simulink model "PI_for_pumps_test"  (R2020a)
settings: Solver=FixedStepAuto  StartTime=0.0  StopTime=inf  FixedStep=1  RelTol=1e-3
libraries: modbusMatLib x6, simulink x4, realtime_pacer_lib x1
settings Model: Creator=pppc  LastModifiedBy=adish
settings DebuggingCC: InheritedTsInSrcMsg=none
settings SFSimCC: CustomCodeUndefinedFunction=UseInterfaceOnly

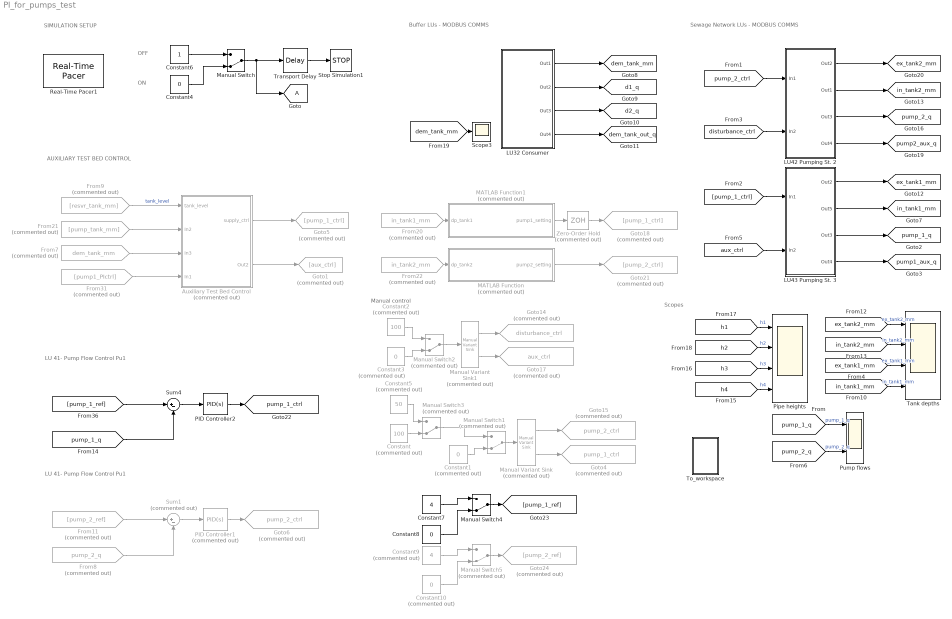
== system PI_for_pumps_test ==
  note: ON
  note: AUXILIARY TEST BED CONTROL
  note: OFF
  note: SIMULATION SETUP
  note: LU 41- Pump Flow Control Pu1
  note: Buffer LUs - MODBUS COMMS
  note: Sewage Network LUs - MODBUS COMMS
  note: Manual control
  note: Scopes
  note: LU 41- Pump Flow Control Pu1
  "Auxiliary Test Bed Control " : Subsystem  Commented=on
  Constant : Constant  Commented=on  Value=100
  Constant1 : Constant  Commented=on  Value=0
  Constant10 : Constant  Commented=on  Value=0
  Constant2 : Constant  Commented=on  Value=100
  Constant3 : Constant  Commented=on  Value=0
  Constant4 : Constant  Value=0
  Constant5 : Constant  Commented=on  Value=50
  Constant6 : Constant
  Constant7 : Constant  Value=4
  Constant8 : Constant  Value=0
  Constant9 : Constant  Commented=on  Value=4
  From11 : From  Commented=on  GotoTag=pump_2_ref
  From20 : From  Commented=on  GotoTag=in_tank1_mm  TagVisibility=global
  From21 : From  Commented=on  GotoTag=pump_tank_mm  TagVisibility=global
  From22 : From  Commented=on  GotoTag=in_tank2_mm  TagVisibility=global
  From31 : From  Commented=on  GotoTag=pump1_PIctrl  TagVisibility=global
  From7 : From  Commented=on  GotoTag=dem_tank_mm  TagVisibility=global
  From8 : From  Commented=on  GotoTag=pump_2_q  TagVisibility=global
  From9 : From  Commented=on  GotoTag=resvr_tank_mm  TagVisibility=global
  Goto1 : Goto  Commented=on  GotoTag=aux_ctrl
  Goto14 : Goto  Commented=on  GotoTag=disturbance_ctrl  TagVisibility=global
  Goto15 : Goto  Commented=on  GotoTag=pump_2_ctrl  TagVisibility=global
  Goto17 : Goto  Commented=on  GotoTag=aux_ctrl  TagVisibility=global
  Goto18 : Goto  Commented=on  GotoTag=pump_1_ctrl
  Goto21 : Goto  Commented=on  GotoTag=pump_2_ctrl
  Goto24 : Goto  Commented=on  GotoTag=pump_2_ref
  Goto4 : Goto  Commented=on  GotoTag=pump_1_ctrl  TagVisibility=global
  Goto5 : Goto  Commented=on  GotoTag=pump_1_ctrl
  Goto6 : Goto  Commented=on  GotoTag=pump_2_ctrl  TagVisibility=global
  LU32 Consumer : Subsystem
  LU42 Pumping St. 2 : Subsystem
  LU43 Pumping St. 3 : Subsystem
  MATLAB Function : MATLAB Function  Commented=on  TreatAsAtomicUnit=on
  MATLAB Function1 : MATLAB Function  Commented=on  TreatAsAtomicUnit=on
  Manual Variant Sink : simulink/Signal Routing/Manual Variant Sink  Commented=on  NumChoices=2  LabelModeActiveChoice=V_2
  Manual Variant Sink1 : simulink/Signal Routing/Manual Variant Sink  Commented=on  NumChoices=2  LabelModeActiveChoice=V_2
  Manual Switch : ManualSwitch  CurrentSetting=0
  Manual Switch{1..3,5} (4 alike) : ManualSwitch  Commented=on  CurrentSetting=0
  Manual Switch4 : ManualSwitch  CurrentSetting=0
  PID Controller1 : simulink/Continuous/PID Controller  Commented=on  Controller=PID  Form=Parallel  TimeDomain=Continuous-time  UseExternalTs=off  SampleTime=1  IntegratorMethod=Forward Euler  FilterMethod=Forward Euler  ControllerParametersSource=internal  P=7.4309  I=30.1148  D=0  UseFilter=on  N=100  TunerSelectOption=Transfer Function Based (PID Tuner App)  InitialConditionSource=internal  InitialConditionForIntegrator=0  InitialConditionForFilter=0  DifferentiatorICPrevScaledInput=0  ExternalReset=none  TrackingMode=off  Kt=1  LimitOutput=on  UpperSaturationLimit=95  LowerSaturationLimit=10  LinearizeAsGain=off  AntiWindupMode=clamping  Kb=1  POutMin=[]  POutMax=[]  IOutMin=[]  IOutMax=[]  DOutMin=[]  DOutMax=[]  NOutMin=[]  NOutMax=[]  SumOutMin=[]  SumOutMax=[]  SaturationOutMin=[]  SaturationOutMax=[]  PParamMin=[]  PParamMax=[]  IParamMin=[]  IParamMax=[]  DParamMin=[]  DParamMax=[]  NParamMin=[]  NParamMax=[]  KbParamMin=[]  KbParamMax=[]  KtParamMin=[]  KtParamMax=[]  KbOutMin=[]  KbOutMax=[]  KtOutMin=[]  KtOutMax=[]  IntegratorOutMin=[]  IntegratorOutMax=[]  FilterOutMin=[]  FilterOutMax=[]  SumI1OutMin=[]  SumI1OutMax=[]  SumI2OutMin=[]  SumI2OutMax=[]  SumI3OutMin=[]  SumI3OutMax=[]  SumI4OutMin=[]  SumI4OutMax=[]  SumDOutMin=[]  SumDOutMax=[]  DifferentiatorOutMin=[]  DifferentiatorOutMax=[]  FilterDiffOutCoefMin=[]  FilterDiffOutCoefMax=[]  ReciprocalOutMin=[]  ReciprocalOutMax=[]  SumDenOutMin=[]  SumDenOutMax=[]  SumNumOutMin=[]  SumNumOutMax=[]  DivideOutMin=[]  DivideOutMax=[]  UdiffTsProdOutMin=[]  UdiffTsProdOutMax=[]  NTsProdOutMin=[]  NTsProdOutMax=[]  UintegralTsProdOutMin=[]  UintegralTsProdOutMax=[]  UngainTsProdOutMin=[]  UngainTsProdOutMax=[]  IntegratorContinuousStateAttributes=''  IntegratorStateMustResolveToSignalObject=off  IntegratorRTWStateStorageClass=Auto  FilterContinuousStateAttributes=''  FilterStateMustResolveToSignalObject=off  FilterRTWStateStorageClass=Auto  ParallelPVariant=InternalParameters  IdealPVariant=Disabled  IVariant=InternalParameters  DVariant=InternalParameters  IntegratorVariant=Continuous  SatVariant=Enabled  AWVariant=ContClampingParallel  PCopyVariant=Disabled  TRVariant=Disabled  FdbkBlocksVariant=Forward  IdealPFdbkVariant=Disabled  SatFdbkVariant=Disabled  DerivativeFilterVariant=ContFilter  NVariant=InternalParameters  NCopyVariant=Disabled  FilterICVariant=InternalICsFilter  IntegratorICVariant=InternalICs  ExternalResetVariant=Disabled  TRSumVariant=Passthrough  SumFdbkVariant=Disabled  SumVariant=Sum_PID  TsampFilterVariant=InternalTs  TsampNgainVariant=Passthrough  TsampIntegralVariant=Passthrough
  PID Controller2 : simulink/Continuous/PID Controller  Controller=PID  Form=Parallel  TimeDomain=Continuous-time  UseExternalTs=off  SampleTime=1  IntegratorMethod=Forward Euler  FilterMethod=Forward Euler  ControllerParametersSource=internal  P=7.4309  I=30.1148  D=0  UseFilter=on  N=100  TunerSelectOption=Transfer Function Based (PID Tuner App)  InitialConditionSource=internal  InitialConditionForIntegrator=0  InitialConditionForFilter=0  DifferentiatorICPrevScaledInput=0  ExternalReset=none  TrackingMode=off  Kt=1  LimitOutput=on  UpperSaturationLimit=95  LowerSaturationLimit=10  LinearizeAsGain=off  AntiWindupMode=clamping  Kb=1  POutMin=[]  POutMax=[]  IOutMin=[]  IOutMax=[]  DOutMin=[]  DOutMax=[]  NOutMin=[]  NOutMax=[]  SumOutMin=[]  SumOutMax=[]  SaturationOutMin=[]  SaturationOutMax=[]  PParamMin=[]  PParamMax=[]  IParamMin=[]  IParamMax=[]  DParamMin=[]  DParamMax=[]  NParamMin=[]  NParamMax=[]  KbParamMin=[]  KbParamMax=[]  KtParamMin=[]  KtParamMax=[]  KbOutMin=[]  KbOutMax=[]  KtOutMin=[]  KtOutMax=[]  IntegratorOutMin=[]  IntegratorOutMax=[]  FilterOutMin=[]  FilterOutMax=[]  SumI1OutMin=[]  SumI1OutMax=[]  SumI2OutMin=[]  SumI2OutMax=[]  SumI3OutMin=[]  SumI3OutMax=[]  SumI4OutMin=[]  SumI4OutMax=[]  SumDOutMin=[]  SumDOutMax=[]  DifferentiatorOutMin=[]  DifferentiatorOutMax=[]  FilterDiffOutCoefMin=[]  FilterDiffOutCoefMax=[]  ReciprocalOutMin=[]  ReciprocalOutMax=[]  SumDenOutMin=[]  SumDenOutMax=[]  SumNumOutMin=[]  SumNumOutMax=[]  DivideOutMin=[]  DivideOutMax=[]  UdiffTsProdOutMin=[]  UdiffTsProdOutMax=[]  NTsProdOutMin=[]  NTsProdOutMax=[]  UintegralTsProdOutMin=[]  UintegralTsProdOutMax=[]  UngainTsProdOutMin=[]  UngainTsProdOutMax=[]  IntegratorContinuousStateAttributes=''  IntegratorStateMustResolveToSignalObject=off  IntegratorRTWStateStorageClass=Auto  FilterContinuousStateAttributes=''  FilterStateMustResolveToSignalObject=off  FilterRTWStateStorageClass=Auto  ParallelPVariant=InternalParameters  IdealPVariant=Disabled  IVariant=InternalParameters  DVariant=InternalParameters  IntegratorVariant=Continuous  SatVariant=Enabled  AWVariant=ContClampingParallel  PCopyVariant=Disabled  TRVariant=Disabled  FdbkBlocksVariant=Forward  IdealPFdbkVariant=Disabled  SatFdbkVariant=Disabled  DerivativeFilterVariant=ContFilter  NVariant=InternalParameters  NCopyVariant=Disabled  FilterICVariant=InternalICsFilter  IntegratorICVariant=InternalICs  ExternalResetVariant=Disabled  TRSumVariant=Passthrough  SumFdbkVariant=Disabled  SumVariant=Sum_PID  TsampFilterVariant=InternalTs  TsampNgainVariant=Passthrough  TsampIntegralVariant=Passthrough
  Pipe heights : Scope  NumInputPorts=4
  Pump flows : Scope  NumInputPorts=2
  Real-Time Pacer1 : realtime_pacer_lib/Real-Time Pacer  simTimePerRealTime=1
  Scope3 : Scope
  Stop Simulation1 : Stop
  Sum1 : Sum  Commented=on  Inputs=|+-
  Sum4 : Sum  Inputs=|+-
  Tank depths : Scope  NumInputPorts=4
  To_workspace : Subsystem
  Transport Delay : TransportDelay  DelayTime=2
  Zero-Order Hold : ZeroOrderHold  Commented=on  SampleTime=4
  tag scope: A=global, d1_q=global, d2_q=global, dem_tank_mm=global, dem_tank_out_q=global, ex_tank1_mm=global, ex_tank2_mm=global, in_tank1_mm=global, in_tank2_mm=global, pump1_aux_q=global, pump2_aux_q=global, pump_1_ctrl=global, pump_1_q=global, pump_2_q=global
  wires:
  Manual Switch/1 -> [A], Transport Delay/1
  Transport Delay/1 -> Stop Simulation1/1
  Constant6/1 -> Manual Switch/1
  Constant4/1 -> Manual Switch/2
  From9/1 -> "Auxiliary Test Bed Control "/1(tank_level)  "tank_level"
  From21/1 -> "Auxiliary Test Bed Control "/2(In2)
  From7/1 -> "Auxiliary Test Bed Control "/3(In3)
  "Auxiliary Test Bed Control "/1(supply_ctrl) -> Goto5/1
  "Auxiliary Test Bed Control "/2(Out2) -> Goto1/1
  LU32 Consumer/1(Out1) -> [dem_tank_mm]
  LU32 Consumer/2(Out2) -> [d1_q]
  LU32 Consumer/3(Out3) -> [d2_q]
  LU32 Consumer/4(Out4) -> [dem_tank_out_q]
  [pump_1_ref] -> Sum4/1
  [pump_1_q] -> Sum4/2
  Sum4/1 -> PID Controller2/1
  From31/1 -> "Auxiliary Test Bed Control "/4(In1)
  [pump_2_ctrl] -> LU42 Pumping St. 2/1(In1)
  LU42 Pumping St. 2/4(Out4) -> [pump2_aux_q]
  LU42 Pumping St. 2/1(Out2) -> [ex_tank2_mm]
  LU42 Pumping St. 2/3(Out3) -> [pump_2_q]
  [disturbance_ctrl] -> LU42 Pumping St. 2/2(In2)
  [aux_ctrl] -> LU43 Pumping St. 3/2(In2)
  LU43 Pumping St. 3/3(Out3) -> [pump_1_q]
  LU43 Pumping St. 3/4(Out4) -> [pump1_aux_q]
  [pump_1_ctrl] -> LU43 Pumping St. 3/1(In1)
  LU43 Pumping St. 3/1(Out2) -> [ex_tank1_mm]
  LU43 Pumping St. 3/2(Out5) -> [in_tank1_mm]
  Constant1/1 -> Manual Switch1/2
  Constant3/1 -> Manual Switch2/2
  Constant2/1 -> Manual Switch2/1
  Constant/1 -> Manual Switch3/2
  Constant5/1 -> Manual Switch3/1
  Manual Switch3/1 -> Manual Switch1/1
  LU42 Pumping St. 2/2(Out1) -> [in_tank2_mm]
  [in_tank2_mm] -> Tank depths/2  "in_tank2_mm"
  [ex_tank2_mm] -> Tank depths/1  "ex_tank2_mm"
  Manual Switch1/1 -> Manual Variant Sink/1
  Manual Variant Sink/1 -> Goto15/1
  Manual Variant Sink/2 -> Goto4/1
  Manual Switch2/1 -> Manual Variant Sink1/1
  Manual Variant Sink1/1 -> Goto14/1
  Manual Variant Sink1/2 -> Goto17/1
  [h1] -> Pipe heights/1  "h1"
  [h2] -> Pipe heights/2  "h2"
  [h4] -> Pipe heights/4  "h4"
  [h3] -> Pipe heights/3  "h3"
  [dem_tank_mm] -> Scope3/1
  MATLAB Function1/1(pump1_setting) -> Zero-Order Hold/1
  From20/1 -> MATLAB Function1/1(dp_tank1)
  Zero-Order Hold/1 -> Goto18/1
  From22/1 -> MATLAB Function/1(dp_tank2)
  MATLAB Function/1(pump2_setting) -> Goto21/1
  [ex_tank1_mm] -> Tank depths/3  "ex_tank1_mm"
  [in_tank1_mm] -> Tank depths/4  "in_tank1_mm"
  [pump_1_q] -> Pump flows/1  "pump_1_q"
  [pump_2_q] -> Pump flows/2  "pump_2_q"
  PID Controller2/1 -> [pump_1_ctrl]
  PID Controller1/1 -> Goto6/1
  Sum1/1 -> PID Controller1/1
  From8/1 -> Sum1/2
  From11/1 -> Sum1/1
  Manual Switch4/1 -> [pump_1_ref]
  Constant7/1 -> Manual Switch4/1
  Constant8/1 -> Manual Switch4/2
  Constant10/1 -> Manual Switch5/2
  Constant9/1 -> Manual Switch5/1
  Manual Switch5/1 -> Goto24/1

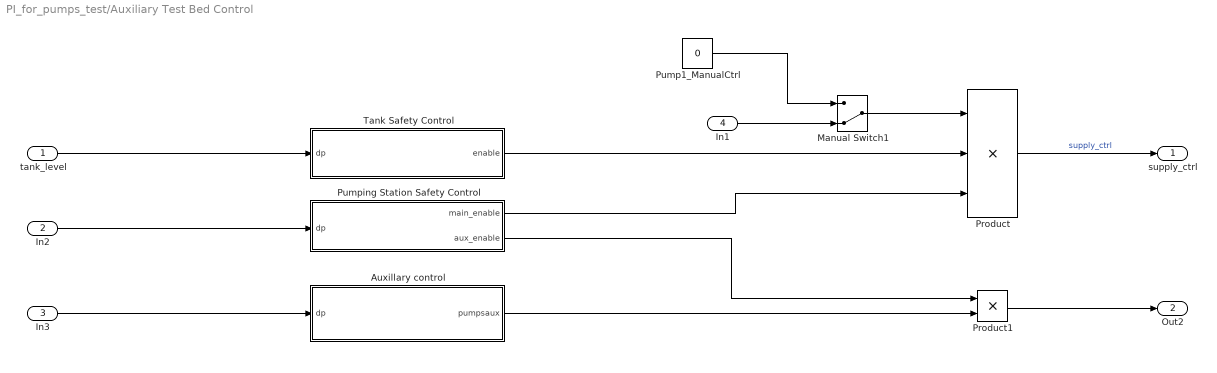
== system PI_for_pumps_test/Auxiliary Test Bed Control  ==
  tank_level : Inport
  In2 : Inport  Port=2
  In3 : Inport  Port=3
  In1 : Inport  Port=4
  Auxillary control : MATLAB Function  TreatAsAtomicUnit=on
  Manual Switch1 : ManualSwitch  CurrentSetting=0
  Product : Product  Inputs=3
  Product1 : Product
  Pump1_ManualCtrl : Constant  Value=0
  Pumping Station Safety Control : MATLAB Function  TreatAsAtomicUnit=on
  Tank Safety Control : MATLAB Function  TreatAsAtomicUnit=on
  supply_ctrl : Outport  VectorParamsAs1DForOutWhenUnconnected=off
  Out2 : Outport  Port=2  VectorParamsAs1DForOutWhenUnconnected=off
  wires:
  Pumping Station Safety Control/1(main_enable) -> Product/3
  Pump1_ManualCtrl/1 -> Manual Switch1/1
  Auxillary control/1(pumpsaux) -> Product1/2
  Tank Safety Control/1(enable) -> Product/2
  Pumping Station Safety Control/2(aux_enable) -> Product1/1
  Manual Switch1/1 -> Product/1
  Product1/1 -> Out2/1
  tank_level/1 -> Tank Safety Control/1(dp)
  In3/1 -> Auxillary control/1(dp)
  Product/1 -> supply_ctrl/1  "supply_ctrl"
  In2/1 -> Pumping Station Safety Control/1(dp)
  In1/1 -> Manual Switch1/2

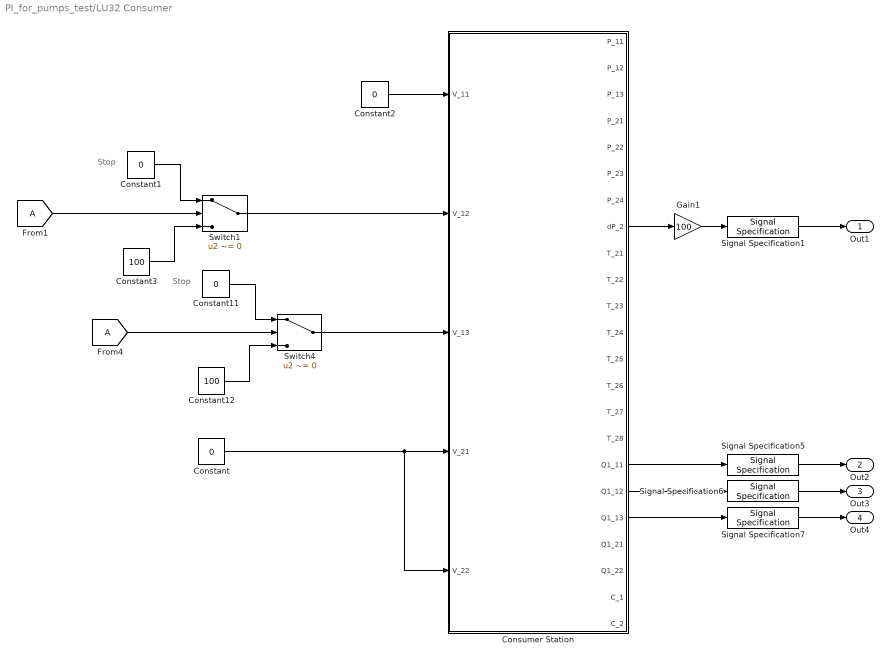
== system PI_for_pumps_test/LU32 Consumer ==
  note: Stop
  note: Stop
  Constant{,1..2,11} (4 alike) : Constant  Value=0
  Constant12 : Constant  Value=100
  Constant3 : Constant  Value=100
  Consumer Station : Subsystem
  Gain1 : Gain  Gain=100
  Signal Specification1 : SignalSpecification  Unit=mm
  Signal Specification5 : SignalSpecification  Unit=l/min
  Signal Specification6 : SignalSpecification  Unit=l/min
  Signal Specification7 : SignalSpecification  Unit=l/min
  Switch1 : Switch  Criteria=u2 ~= 0
  Switch4 : Switch  Criteria=u2 ~= 0
  Out1 : Outport  VectorParamsAs1DForOutWhenUnconnected=off
  Out2 : Outport  Port=2  VectorParamsAs1DForOutWhenUnconnected=off
  Out3 : Outport  Port=3  VectorParamsAs1DForOutWhenUnconnected=off
  Out4 : Outport  Port=4  VectorParamsAs1DForOutWhenUnconnected=off
  wires:
  Consumer Station/8(dP_2) -> Gain1/1
  Switch4/1 -> Consumer Station/3(V_13)
  Consumer Station/19(Q1_13) -> Signal Specification7/1
  Constant12/1 -> Switch4/3
  Consumer Station/17(Q1_11) -> Signal Specification5/1
  Consumer Station/18(Q1_12) -> Signal Specification6/1
  Gain1/1 -> Signal Specification1/1
  [A] -> Switch4/2
  Signal Specification7/1 -> Out4/1
  Constant11/1 -> Switch4/1
  Signal Specification5/1 -> Out2/1
  Constant/1 -> Consumer Station/5(V_22), Consumer Station/4(V_21)
  Signal Specification6/1 -> Out3/1
  Signal Specification1/1 -> Out1/1
  Constant1/1 -> Switch1/1
  [A] -> Switch1/2
  Constant3/1 -> Switch1/3
  Switch1/1 -> Consumer Station/2(V_12)
  Constant2/1 -> Consumer Station/1(V_11)

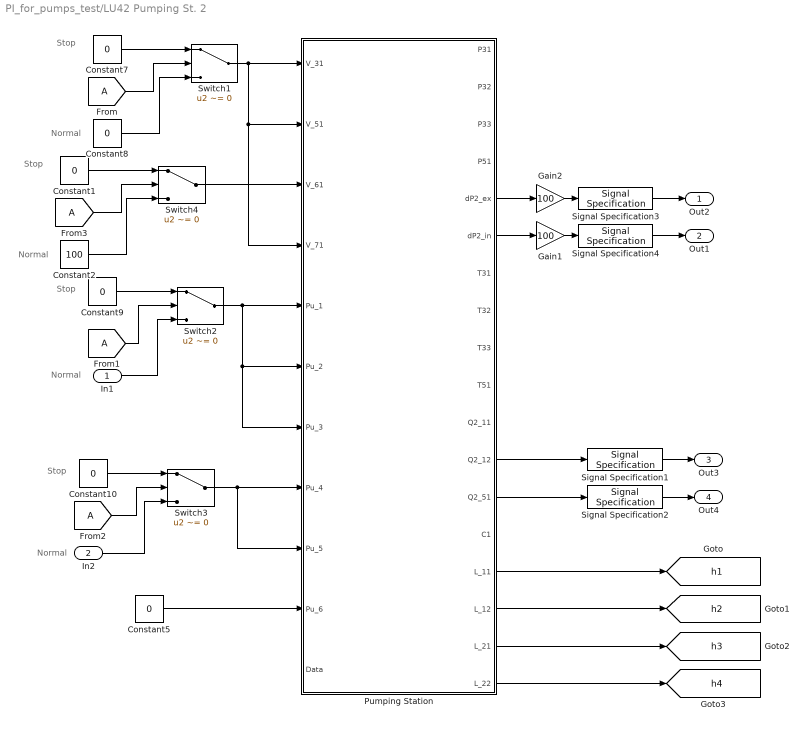
== system PI_for_pumps_test/LU42 Pumping St. 2 ==
  note: Stop
  note: Stop
  note: Normal
  note: Stop
  note: Normal
  note: Normal
  note: Stop
  note: Normal
  In1 : Inport
  In2 : Inport  Port=2
  Constant{1,5,7..10} (6 alike) : Constant  Value=0
  Constant2 : Constant  Value=100
  Gain1 : Gain  Gain=100
  Gain2 : Gain  Gain=100
  Pumping Station : Subsystem
  Signal Specification1 : SignalSpecification  Unit=l/min
  Signal Specification2 : SignalSpecification  Unit=l/min
  Signal Specification3 : SignalSpecification  Unit=mm
  Signal Specification4 : SignalSpecification  Unit=mm
  Switch{1..4} (4 alike) : Switch  Criteria=u2 ~= 0
  Out2 : Outport  VectorParamsAs1DForOutWhenUnconnected=off
  Out1 : Outport  Port=2  VectorParamsAs1DForOutWhenUnconnected=off
  Out3 : Outport  Port=3  VectorParamsAs1DForOutWhenUnconnected=off
  Out4 : Outport  Port=4  VectorParamsAs1DForOutWhenUnconnected=off
  tag scope: h1=global, h2=global, h3=global, h4=global
  wires:
  Switch2/1 -> Pumping Station/7(Pu_3), Pumping Station/6(Pu_2), Pumping Station/5(Pu_1)
  [A] -> Switch1/2
  Constant7/1 -> Switch1/1
  Constant8/1 -> Switch1/3
  Switch3/1 -> Pumping Station/9(Pu_5), Pumping Station/8(Pu_4)
  Constant10/1 -> Switch3/1
  In1/1 -> Switch2/3
  [A] -> Switch2/2
  Constant9/1 -> Switch2/1
  In2/1 -> Switch3/3
  Gain2/1 -> Signal Specification3/1
  Constant5/1 -> Pumping Station/10(Pu_6)
  Signal Specification3/1 -> Out2/1
  [A] -> Switch3/2
  Pumping Station/5(dP2_ex) -> Gain2/1
  Switch1/1 -> Pumping Station/4(V_71), Pumping Station/2(V_51), Pumping Station/1(V_31)
  Signal Specification1/1 -> Out3/1
  Signal Specification2/1 -> Out4/1
  Pumping Station/12(Q2_12) -> Signal Specification1/1
  Pumping Station/13(Q2_51) -> Signal Specification2/1
  Pumping Station/6(dP2_in) -> Gain1/1
  Gain1/1 -> Signal Specification4/1
  Signal Specification4/1 -> Out1/1
  Pumping Station/15(L_11) -> [h1]
  Pumping Station/16(L_12) -> [h2]
  Pumping Station/17(L_21) -> [h3]
  Pumping Station/18(L_22) -> [h4]
  Constant1/1 -> Switch4/1
  Constant2/1 -> Switch4/3
  [A] -> Switch4/2
  Switch4/1 -> Pumping Station/3(V_61)

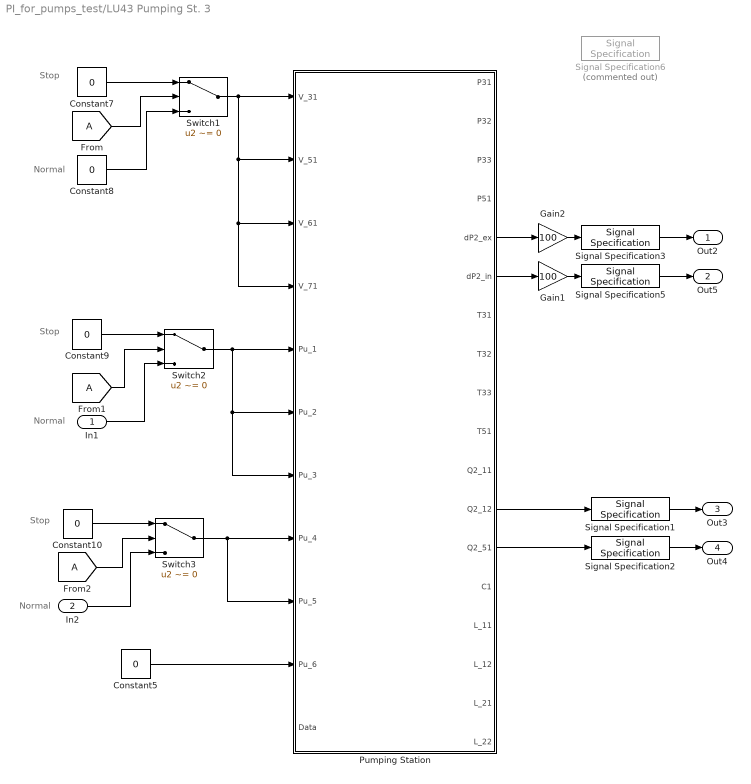
== system PI_for_pumps_test/LU43 Pumping St. 3 ==
  note: Stop
  note: Stop
  note: Normal
  note: Stop
  note: Normal
  note: Normal
  In1 : Inport
  In2 : Inport  Port=2
  Constant{5,7..10} (5 alike) : Constant  Value=0
  Gain1 : Gain  Gain=100
  Gain2 : Gain  Gain=100
  Pumping Station : Subsystem
  Signal Specification1 : SignalSpecification  Unit=l/min
  Signal Specification2 : SignalSpecification  Unit=l/min
  Signal Specification3 : SignalSpecification  Unit=mm
  Signal Specification5 : SignalSpecification  Unit=mm
  Signal Specification6 : SignalSpecification  Commented=on  Unit=bar
  Switch1 : Switch  Criteria=u2 ~= 0
  Switch2 : Switch  Criteria=u2 ~= 0
  Switch3 : Switch  Criteria=u2 ~= 0
  Out2 : Outport  VectorParamsAs1DForOutWhenUnconnected=off
  Out5 : Outport  Port=2  VectorParamsAs1DForOutWhenUnconnected=off
  Out3 : Outport  Port=3  VectorParamsAs1DForOutWhenUnconnected=off
  Out4 : Outport  Port=4  VectorParamsAs1DForOutWhenUnconnected=off
  wires:
  Switch2/1 -> Pumping Station/7(Pu_3), Pumping Station/6(Pu_2), Pumping Station/5(Pu_1)
  [A] -> Switch1/2
  Constant7/1 -> Switch1/1
  Constant8/1 -> Switch1/3
  Switch3/1 -> Pumping Station/9(Pu_5), Pumping Station/8(Pu_4)
  Constant10/1 -> Switch3/1
  In1/1 -> Switch2/3
  [A] -> Switch2/2
  Constant9/1 -> Switch2/1
  In2/1 -> Switch3/3
  Gain2/1 -> Signal Specification3/1
  Constant5/1 -> Pumping Station/10(Pu_6)
  Signal Specification3/1 -> Out2/1
  [A] -> Switch3/2
  Pumping Station/5(dP2_ex) -> Gain2/1
  Switch1/1 -> Pumping Station/4(V_71), Pumping Station/3(V_61), Pumping Station/2(V_51), Pumping Station/1(V_31)
  Signal Specification1/1 -> Out3/1
  Signal Specification2/1 -> Out4/1
  Pumping Station/12(Q2_12) -> Signal Specification1/1
  Pumping Station/13(Q2_51) -> Signal Specification2/1
  Pumping Station/6(dP2_in) -> Gain1/1
  Signal Specification5/1 -> Out5/1
  Gain1/1 -> Signal Specification5/1

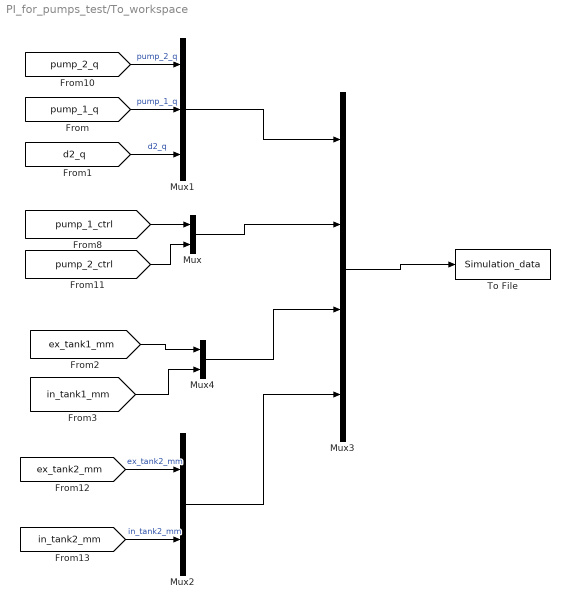
== system PI_for_pumps_test/To_workspace ==
  Mux : Mux  Inputs=2
  Mux1 : Mux  Inputs=3
  Mux2 : Mux  Inputs=2
  Mux3 : Mux
  Mux4 : Mux  Inputs=2
  To File : ToFile  Filename=Simulation_data  SaveFormat=Timeseries
  wires:
  [pump_2_q] -> Mux1/1  "pump_2_q"
  [in_tank2_mm] -> Mux2/2  "in_tank2_mm"
  [ex_tank2_mm] -> Mux2/1  "ex_tank2_mm"
  [pump_1_q] -> Mux1/2  "pump_1_q"
  [d2_q] -> Mux1/3  "d2_q"
  Mux1/1 -> Mux3/1
  Mux3/1 -> To File/1
  [pump_1_ctrl] -> Mux/1
  [pump_2_ctrl] -> Mux/2
  Mux/1 -> Mux3/2
  Mux2/1 -> Mux3/4
  [ex_tank1_mm] -> Mux4/1
  [in_tank1_mm] -> Mux4/2
  Mux4/1 -> Mux3/3

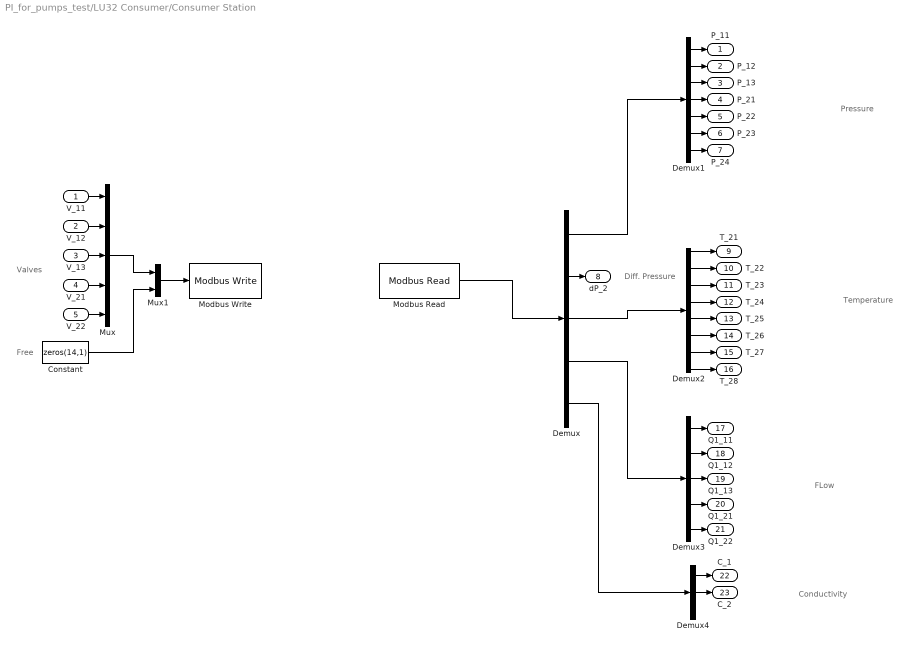
== system PI_for_pumps_test/LU32 Consumer/Consumer Station ==
  note: Pressure
  note: Temperature
  note: FLow
  note: Conductivity
  note: Valves
  note: Diff. Pressure
  note: Free
  V_11 : Inport
  V_12 : Inport  Port=2
  V_13 : Inport  Port=3
  V_21 : Inport  Port=4
  V_22 : Inport  Port=5
  Constant : Constant  Value=zeros(14,1)
  Demux : Demux  Outputs=[7 1 8 5 3]
  Demux1 : Demux  Outputs=7
  Demux2 : Demux  Outputs=8
  Demux3 : Demux  Outputs=5
  Demux4 : Demux  Outputs=3
  Modbus Read : modbusMatLib/Modbus Read  registry=0  ipAddress='192.168.100.32'  port=502
  Modbus Write : modbusMatLib/Modbus Write  registry=001  port=502  ipAddress='192.168.100.32'
  Mux : Mux  Inputs=5
  Mux1 : Mux  Inputs=2
  P_11 : Outport  VectorParamsAs1DForOutWhenUnconnected=off
  P_12 : Outport  Port=2  VectorParamsAs1DForOutWhenUnconnected=off
  P_13 : Outport  Port=3  VectorParamsAs1DForOutWhenUnconnected=off
  P_21 : Outport  Port=4  VectorParamsAs1DForOutWhenUnconnected=off
  P_22 : Outport  Port=5  VectorParamsAs1DForOutWhenUnconnected=off
  P_23 : Outport  Port=6  VectorParamsAs1DForOutWhenUnconnected=off
  P_24 : Outport  Port=7  VectorParamsAs1DForOutWhenUnconnected=off
  dP_2 : Outport  Port=8  VectorParamsAs1DForOutWhenUnconnected=off
  T_21 : Outport  Port=9  VectorParamsAs1DForOutWhenUnconnected=off
  T_22 : Outport  Port=10  VectorParamsAs1DForOutWhenUnconnected=off
  T_23 : Outport  Port=11  VectorParamsAs1DForOutWhenUnconnected=off
  T_24 : Outport  Port=12  VectorParamsAs1DForOutWhenUnconnected=off
  T_25 : Outport  Port=13  VectorParamsAs1DForOutWhenUnconnected=off
  T_26 : Outport  Port=14  VectorParamsAs1DForOutWhenUnconnected=off
  T_27 : Outport  Port=15  VectorParamsAs1DForOutWhenUnconnected=off
  T_28 : Outport  Port=16  VectorParamsAs1DForOutWhenUnconnected=off
  Q1_11 : Outport  Port=17  VectorParamsAs1DForOutWhenUnconnected=off
  Q1_12 : Outport  Port=18  VectorParamsAs1DForOutWhenUnconnected=off
  Q1_13 : Outport  Port=19  VectorParamsAs1DForOutWhenUnconnected=off
  Q1_21 : Outport  Port=20  VectorParamsAs1DForOutWhenUnconnected=off
  Q1_22 : Outport  Port=21  VectorParamsAs1DForOutWhenUnconnected=off
  C_1 : Outport  Port=22  VectorParamsAs1DForOutWhenUnconnected=off
  C_2 : Outport  Port=23  VectorParamsAs1DForOutWhenUnconnected=off
  wires:
  Mux/1 -> Mux1/1
  Mux1/1 -> Modbus Write/1
  Constant/1 -> Mux1/2
  Demux1/5 -> P_22/1
  V_12/1 -> Mux/2
  Demux1/6 -> P_23/1
  Demux1/3 -> P_13/1
  Demux1/4 -> P_21/1
  V_13/1 -> Mux/3
  Demux3/2 -> Q1_12/1
  Demux3/5 -> Q1_22/1
  Demux/2 -> dP_2/1
  Demux3/1 -> Q1_11/1
  Demux1/2 -> P_12/1
  Demux2/5 -> T_25/1
  Demux4/1 -> C_1/1
  V_21/1 -> Mux/4
  Demux3/3 -> Q1_13/1
  Demux1/1 -> P_11/1
  Demux3/4 -> Q1_21/1
  V_11/1 -> Mux/1
  Demux2/4 -> T_24/1
  Demux2/3 -> T_23/1
  Demux2/2 -> T_22/1
  Demux2/1 -> T_21/1
  Demux1/7 -> P_24/1
  V_22/1 -> Mux/5
  Demux2/7 -> T_27/1
  Demux/5 -> Demux4/1
  Demux/1 -> Demux1/1
  Demux2/8 -> T_28/1
  Demux4/2 -> C_2/1
  Demux/3 -> Demux2/1
  Demux/4 -> Demux3/1
  Modbus Read/1 -> Demux/1
  Demux2/6 -> T_26/1

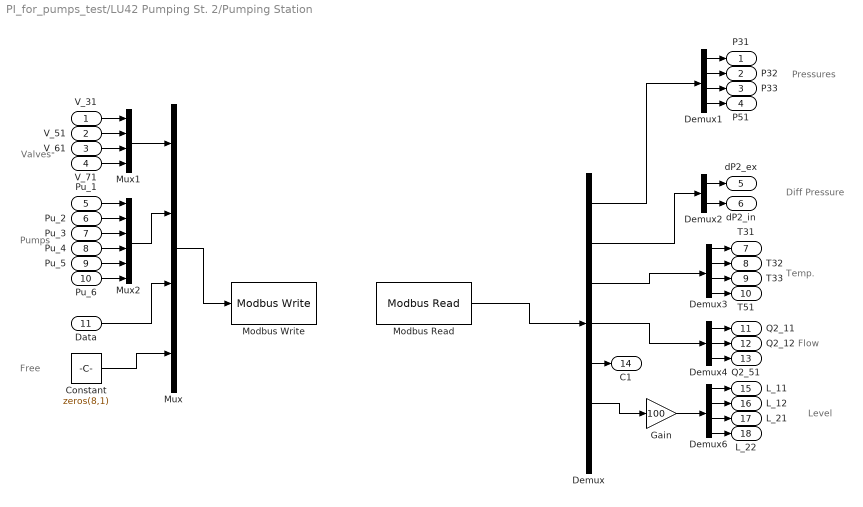
== system PI_for_pumps_test/LU42 Pumping St. 2/Pumping Station ==
  note: Free
  note: Pumps
  note: Valves
  note: Flow
  note: Temp.
  note: Diff Pressure
  note: Pressures
  note: Level
  V_31 : Inport
  V_51 : Inport  Port=2
  V_61 : Inport  Port=3
  V_71 : Inport  Port=4
  Pu_1 : Inport  Port=5
  Pu_2 : Inport  Port=6
  Pu_3 : Inport  Port=7
  Pu_4 : Inport  Port=8
  Pu_5 : Inport  Port=9
  Pu_6 : Inport  Port=10
  Data : Inport  Port=11
  Constant : Constant  Value=zeros(8,1)
  Demux : Demux  Outputs=[4 2 4 3 1 4 6]
  Demux1 : Demux
  Demux2 : Demux  Outputs=2
  Demux3 : Demux
  Demux4 : Demux  Outputs=3
  Demux6 : Demux
  Gain : Gain  Gain=100
  Modbus Read : modbusMatLib/Modbus Read  registry=0  ipAddress='192.168.100.42'  port=502
  Modbus Write : modbusMatLib/Modbus Write  registry=001  port=502  ipAddress='192.168.100.42'
  Mux : Mux
  Mux1 : Mux
  Mux2 : Mux  Inputs=6
  P31 : Outport  VectorParamsAs1DForOutWhenUnconnected=off
  P32 : Outport  Port=2  VectorParamsAs1DForOutWhenUnconnected=off
  P33 : Outport  Port=3  VectorParamsAs1DForOutWhenUnconnected=off
  P51 : Outport  Port=4  VectorParamsAs1DForOutWhenUnconnected=off
  dP2_ex : Outport  Port=5  VectorParamsAs1DForOutWhenUnconnected=off
  dP2_in : Outport  Port=6  VectorParamsAs1DForOutWhenUnconnected=off
  T31 : Outport  Port=7  VectorParamsAs1DForOutWhenUnconnected=off
  T32 : Outport  Port=8  VectorParamsAs1DForOutWhenUnconnected=off
  T33 : Outport  Port=9  VectorParamsAs1DForOutWhenUnconnected=off
  T51 : Outport  Port=10  VectorParamsAs1DForOutWhenUnconnected=off
  Q2_11 : Outport  Port=11  VectorParamsAs1DForOutWhenUnconnected=off
  Q2_12 : Outport  Port=12  VectorParamsAs1DForOutWhenUnconnected=off
  Q2_51 : Outport  Port=13  VectorParamsAs1DForOutWhenUnconnected=off
  C1 : Outport  Port=14  VectorParamsAs1DForOutWhenUnconnected=off
  L_11 : Outport  Port=15  VectorParamsAs1DForOutWhenUnconnected=off
  L_12 : Outport  Port=16  VectorParamsAs1DForOutWhenUnconnected=off
  L_21 : Outport  Port=17  VectorParamsAs1DForOutWhenUnconnected=off
  L_22 : Outport  Port=18  VectorParamsAs1DForOutWhenUnconnected=off
  wires:
  Demux4/1 -> Q2_11/1
  Demux/2 -> Demux2/1
  Demux/4 -> Demux4/1
  Demux2/1 -> dP2_ex/1
  Demux/3 -> Demux3/1
  Demux/1 -> Demux1/1
  Demux3/4 -> T51/1
  Demux1/4 -> P51/1
  Demux3/2 -> T32/1
  Modbus Read/1 -> Demux/1
  Demux6/1 -> L_11/1
  Demux6/2 -> L_12/1
  Demux4/3 -> Q2_51/1
  Demux4/2 -> Q2_12/1
  Demux6/3 -> L_21/1
  Demux6/4 -> L_22/1
  Demux3/3 -> T33/1
  Demux1/1 -> P31/1
  Demux1/2 -> P32/1
  Demux/5 -> C1/1
  Demux1/3 -> P33/1
  Demux2/2 -> dP2_in/1
  Demux3/1 -> T31/1
  Mux/1 -> Modbus Write/1
  Mux1/1 -> Mux/1
  V_31/1 -> Mux1/1
  V_51/1 -> Mux1/2
  V_61/1 -> Mux1/3
  V_71/1 -> Mux1/4
  Pu_4/1 -> Mux2/4
  Pu_3/1 -> Mux2/3
  Pu_1/1 -> Mux2/1
  Pu_2/1 -> Mux2/2
  Mux2/1 -> Mux/2
  Pu_5/1 -> Mux2/5
  Pu_6/1 -> Mux2/6
  Data/1 -> Mux/3
  Constant/1 -> Mux/4
  Gain/1 -> Demux6/1
  Demux/6 -> Gain/1

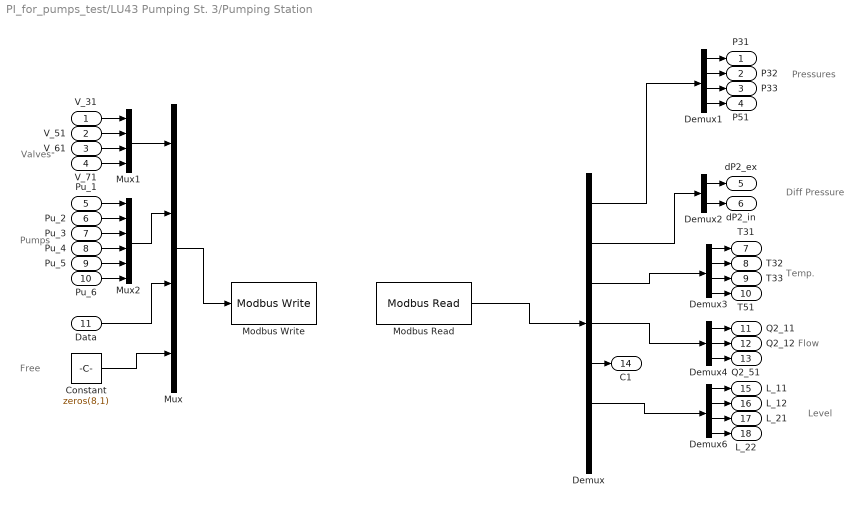
== system PI_for_pumps_test/LU43 Pumping St. 3/Pumping Station ==
  note: Free
  note: Pumps
  note: Valves
  note: Flow
  note: Temp.
  note: Diff Pressure
  note: Pressures
  note: Level
  V_31 : Inport
  V_51 : Inport  Port=2
  V_61 : Inport  Port=3
  V_71 : Inport  Port=4
  Pu_1 : Inport  Port=5
  Pu_2 : Inport  Port=6
  Pu_3 : Inport  Port=7
  Pu_4 : Inport  Port=8
  Pu_5 : Inport  Port=9
  Pu_6 : Inport  Port=10
  Data : Inport  Port=11
  Constant : Constant  Value=zeros(8,1)
  Demux : Demux  Outputs=[4 2 4 3 1 4 6]
  Demux1 : Demux
  Demux2 : Demux  Outputs=2
  Demux3 : Demux
  Demux4 : Demux  Outputs=3
  Demux6 : Demux
  Modbus Read : modbusMatLib/Modbus Read  registry=0  ipAddress='192.168.100.43'  port=502
  Modbus Write : modbusMatLib/Modbus Write  registry=001  port=502  ipAddress='192.168.100.43'
  Mux : Mux
  Mux1 : Mux
  Mux2 : Mux  Inputs=6
  P31 : Outport  VectorParamsAs1DForOutWhenUnconnected=off
  P32 : Outport  Port=2  VectorParamsAs1DForOutWhenUnconnected=off
  P33 : Outport  Port=3  VectorParamsAs1DForOutWhenUnconnected=off
  P51 : Outport  Port=4  VectorParamsAs1DForOutWhenUnconnected=off
  dP2_ex : Outport  Port=5  VectorParamsAs1DForOutWhenUnconnected=off
  dP2_in : Outport  Port=6  VectorParamsAs1DForOutWhenUnconnected=off
  T31 : Outport  Port=7  VectorParamsAs1DForOutWhenUnconnected=off
  T32 : Outport  Port=8  VectorParamsAs1DForOutWhenUnconnected=off
  T33 : Outport  Port=9  VectorParamsAs1DForOutWhenUnconnected=off
  T51 : Outport  Port=10  VectorParamsAs1DForOutWhenUnconnected=off
  Q2_11 : Outport  Port=11  VectorParamsAs1DForOutWhenUnconnected=off
  Q2_12 : Outport  Port=12  VectorParamsAs1DForOutWhenUnconnected=off
  Q2_51 : Outport  Port=13  VectorParamsAs1DForOutWhenUnconnected=off
  C1 : Outport  Port=14  VectorParamsAs1DForOutWhenUnconnected=off
  L_11 : Outport  Port=15  VectorParamsAs1DForOutWhenUnconnected=off
  L_12 : Outport  Port=16  VectorParamsAs1DForOutWhenUnconnected=off
  L_21 : Outport  Port=17  VectorParamsAs1DForOutWhenUnconnected=off
  L_22 : Outport  Port=18  VectorParamsAs1DForOutWhenUnconnected=off
  wires:
  Demux4/1 -> Q2_11/1
  Demux/2 -> Demux2/1
  Demux/4 -> Demux4/1
  Demux2/1 -> dP2_ex/1
  Demux/3 -> Demux3/1
  Demux/6 -> Demux6/1
  Demux/1 -> Demux1/1
  Demux3/4 -> T51/1
  Demux1/4 -> P51/1
  Demux3/2 -> T32/1
  Modbus Read/1 -> Demux/1
  Demux6/1 -> L_11/1
  Demux6/2 -> L_12/1
  Demux4/3 -> Q2_51/1
  Demux4/2 -> Q2_12/1
  Demux6/3 -> L_21/1
  Demux6/4 -> L_22/1
  Demux3/3 -> T33/1
  Demux1/1 -> P31/1
  Demux1/2 -> P32/1
  Demux/5 -> C1/1
  Demux1/3 -> P33/1
  Demux2/2 -> dP2_in/1
  Demux3/1 -> T31/1
  Mux/1 -> Modbus Write/1
  Mux1/1 -> Mux/1
  V_31/1 -> Mux1/1
  V_51/1 -> Mux1/2
  V_61/1 -> Mux1/3
  V_71/1 -> Mux1/4
  Pu_4/1 -> Mux2/4
  Pu_3/1 -> Mux2/3
  Pu_1/1 -> Mux2/1
  Pu_2/1 -> Mux2/2
  Mux2/1 -> Mux/2
  Pu_5/1 -> Mux2/5
  Pu_6/1 -> Mux2/6
  Data/1 -> Mux/3
  Constant/1 -> Mux/4

== matlab function PI_for_pumps_test/MATLAB Function ==
  data: dp_tank2 input; pump2_setting output
function pump2_setting = controller(dp_tank2)

    if dp_tank2<160                       
        pump2_setting=0;                               
    elseif dp_tank2 > 600
        pump2_setting = 100; 
    else
        pump2_setting = 75;
    end
end

== matlab function PI_for_pumps_test/MATLAB Function1 ==
  data: dp_tank1 input; pump1_setting output
function pump1_setting = controller(dp_tank1)
    if dp_tank1<160                       
        pump1_setting=0;
    else
        pump1_setting = round(rand)*75;
    end
end

== matlab function PI_for_pumps_test/Auxiliary Test Bed Control /Tank Safety Control ==
  data: dp input; enable output
function enable = controller(dp)

persistent pumpctrl;        %Create persistent such that previous value of controller can be stored

if isempty(pumpctrl)
    pumpctrl=0;
end


if dp>550                       %Set high limit of level
    enable=0;                    %Stop the pumps if level goes above 'high level' (in mm)
elseif dp<500                   %Set low limit of level
    enable=1;                  %Start the pumps if level goes below 'low level' (in mm)
else
    enable=pumpctrl;         %Run pump as the previous control command
    
end
pumpctrl=enable;             %Update persistent variable
end

== matlab function PI_for_pumps_test/Auxiliary Test Bed Control /Pumping Station Safety Control ==
  settings: updateMethod=DISCRETE
  data: main_enable output; dp input; aux_enable output
function [main_enable,aux_enable] = controller(dp)

persistent aux_pers main_pers;        %Create persistent such that previous value of controller can be stored

if isempty(aux_pers) || isempty(main_pers)
    aux_pers=0;
    main_pers=1;
end


if dp < 90                       %Set low limit of level
    main_enable = 0;            %Stop the pumps if level goes below 'low level' (in mm)
elseif dp > 100
    main_enable = 1;
else
    main_enable = main_pers;
end


if dp > 560                       %Set high limit of level
    aux_enable = 0;               %Stop the pumps if level goes above 'high level' (in mm)
elseif dp < 450
    aux_enable = 1;
else
    aux_enable = aux_pers;
end


aux_pers = aux_enable;             %Update persistent variable
main_pers = main_enable;
end

== matlab function PI_for_pumps_test/Auxiliary Test Bed Control /Auxillary control ==
  data: dp input; pumpsaux output
function pumpsaux = controller(dp)

persistent pumpctrlaux;        %Create persistent such that previous value of controller can be stored

if isempty(pumpctrlaux)
    pumpctrlaux=0;
end


if dp>300                       %Set high limit of level
    pumpsaux=100;                    %Stop the pumps if level goes above 'high level' (in mm)
elseif dp<200                   %Set low limit of level
    pumpsaux=0;                  %Start the pumps if level goes below 'low level' (in mm)
else
    pumpsaux=pumpctrlaux;         %Run pump as the previous control command
    
end
pumpctrlaux=pumpsaux;             %Update persistent variable
end
